simulink model "Diode_Rectifier_Six_Phase_RLload2015"  (R2015b)
settings: Solver=VariableStepAuto  SolverMode=SingleTasking  StartTime=0.0  StopTime=0.04  RelTol=1e-3
undefined symbols (not defined in the file): powergui
libraries: powerlib x24
settings Model: Creator=A.hey  LastModifiedBy=A.hey
settings DataIOCC: LimitDataPoints=off
settings DebuggingCC: AllowSymbolicDim=on  SFUnexpectedBacktrackingDiag=error  SFNoUnconditionalDefaultTransitionDiag=error
settings ModelReferenceCC: PropagateSignalLabelsOutOfModel=on
settings SFSimCC: SimUseLocalCustomCode=on
settings RTWCC: RTWUseLocalCustomCode=on
settings GRTTargetCC: TargetLangStandard=C99 (ISO)
settings ConfigComp: CovMetricSettings=dwe  CovHtmlReporting=off  CovSaveCumulativeToWorkspaceVar=off  CovSaveSingleToWorkspaceVar=off  CovModelRefEnable=Off  CovExternalEMLEnable=on
settings ConfigurationSet: Description=Simscape Multibody

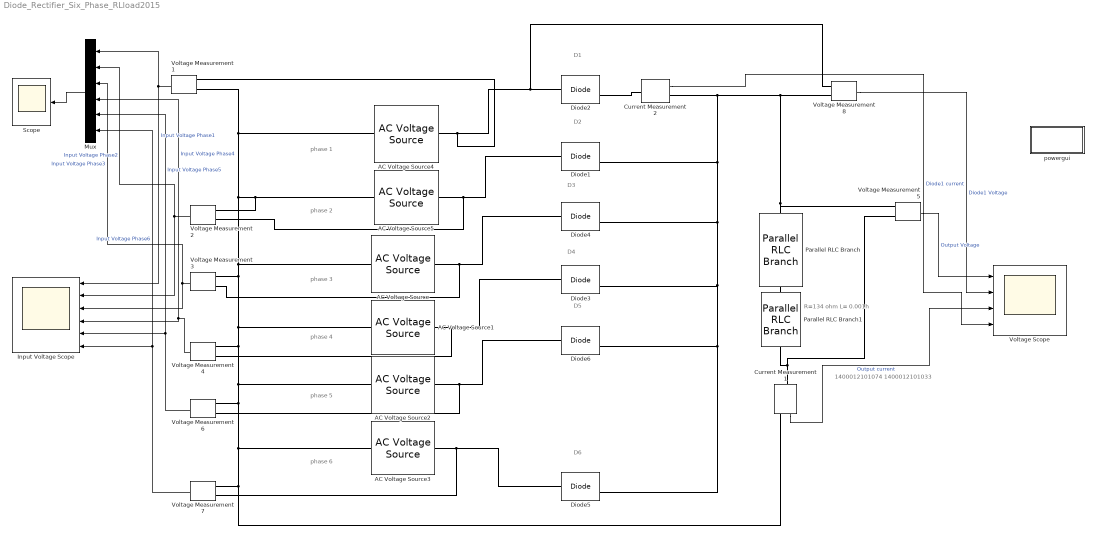
== system Diode_Rectifier_Six_Phase_RLload2015 ==
  note: phase 4
  note: phase 6
  note: phase 1
  note: phase 3
  note: D5
  note: phase 5
  note: D6
  note: D2
  note: phase 2
  note: D1
  note: 1400012101074
      | 1400012101033
  note: D3
  note: D4
  note: R=134 ohm
      | L= 0.001h
  AC Voltage Source : powerlib/Electrical Sources/AC Voltage Source  Amplitude=220  Phase=-180  Frequency=50  SampleTime=0  Measurements=None  BusType=swing  Pref=10e3  Qref=0  Qmin=-inf  Qmax=+inf
  AC Voltage Source1 : powerlib/Electrical Sources/AC Voltage Source  Amplitude=220  Phase=-240  Frequency=50  SampleTime=0  Measurements=None  BusType=swing  Pref=10e3  Qref=0  Qmin=-inf  Qmax=+inf
  AC Voltage Source2 : powerlib/Electrical Sources/AC Voltage Source  Amplitude=220  Phase=-300  Frequency=50  SampleTime=0  Measurements=None  BusType=swing  Pref=10e3  Qref=0  Qmin=-inf  Qmax=+inf
  AC Voltage Source3 : powerlib/Electrical Sources/AC Voltage Source  Amplitude=220  Phase=-360  Frequency=50  SampleTime=0  Measurements=None  BusType=swing  Pref=10e3  Qref=0  Qmin=-inf  Qmax=+inf
  AC Voltage Source4 : powerlib/Electrical Sources/AC Voltage Source  Amplitude=220  Phase=-60  Frequency=50  SampleTime=0  Measurements=None  BusType=swing  Pref=10e3  Qref=0  Qmin=-inf  Qmax=+inf
  AC Voltage Source5 : powerlib/Electrical Sources/AC Voltage Source  Amplitude=220  Phase=-120  Frequency=50  SampleTime=0  Measurements=None  BusType=swing  Pref=10e3  Qref=0  Qmin=-inf  Qmax=+inf
  Current Measurement1 : powerlib/Measurements/Current Measurement  PhasorSimulation=off  OutputType=Complex  PSBequivalent=0
  Current Measurement2 : powerlib/Measurements/Current Measurement  PhasorSimulation=off  OutputType=Complex  PSBequivalent=0
  Diode{1..6} (6 alike) : powerlib/Power Electronics/Diode  Ron=0.001  Lon=0  Vf=0.8  IC=0  UseSnubber=0  Rs=500  Cs=250e-9  Measurements=on
  "Input Voltage Scope " : Scope  NumInputPorts=6
  Mux : Mux  Inputs=6
  Parallel RLC Branch : powerlib/Elements/Parallel RLC Branch  LConnTagsString=a  RConnTagsString=__new0  BranchType=R  Resistance=134  Inductance=1e-3  SetiL0=off  InitialCurrent=0  Capacitance=1e-6  Setx0=off  InitialVoltage=0  Measurements=None
  Parallel RLC Branch1 : powerlib/Elements/Parallel RLC Branch  LConnTagsString=a  RConnTagsString=__new0  BranchType=L  Resistance=134  Inductance=1e-3  SetiL0=off  InitialCurrent=0  Capacitance=1e-6  Setx0=off  InitialVoltage=0  Measurements=None
  Scope : Scope
  Voltage Measurement{1..8} (8 alike) : powerlib/Measurements/Voltage Measurement  PhasorSimulation=off  OutputType=Complex  PSBequivalent=0
  "Voltage Scope " : Scope  NumInputPorts=4
  powergui : Subsystem  Priority=1  AncestorBlock=powerlib/powergui  DialogController=POWERSYS.PowerSysDialog  InitFcn=powergui( 'InitFcn_Callback' , gcb , 0 , [ ] );  mask(PSB option menu block){SimulationMode=Continuous, SampleTime=50e-6, frequency=60, Iterations=50, frequencyindice=50, Pbase=100e6, ErrMax=1e-4, UnitsV=kV, UnitsW=MW, buscounter=0, FunctionMessages=off, echomessages=off, EnableUseOfTLC=off, CurrentSourceSwitches=off, DisableSnubberDevices=off, DisableRonSwitches=off, DisableVfSwitches=off, DisplayEquations=off, SolverType=Tustin/Backward Euler (TBE), Interpol=off, ExternalGateDelay=off, methode=off, Ts=100, x0status=blocks, SPID=on, SwTol=0, HookPort=off, RestoreLinks=warning, ResistiveCurrentMeasurement=off, Frange=[0:2:500], Ylog=off, Xlog=on, ShowGrid=off, save=off, variable=ZData, structure=0, ZoomFFT=off, StartTime=0.0, cycles=1, DisplayStyle=1, fundamental=60, FreqAxis=off, MaxFrequency=1000, frequencyindicesteady=1, RmsSteady=1, display=off}
      mask prompts: SimulationMode "Simulation type:"; SampleTime "Sample time (s):"; frequency "Frequency (Hz):"; Iterations "Max iterations"; frequencyindice "Frequency (Hz)"; Pbase "Base power (VA)"; ErrMax "PQ tolerance (pu)"; UnitsV "Voltage units"; UnitsW "Power units"; buscounter "Load flow bus counter"; FunctionMessages "Disable Specialized Power Systems warnings"; echomessages "Display Specialized Power Systems compilation messages"; EnableUseOfTLC "Use TLC file when in Accelerator Simulation Mode and for code generation"; CurrentSourceSwitches "Disable ideal switching"; DisableSnubberDevices "Disable snubbers in switching devices"; DisableRonSwitches "Disable Ron resistances in switching devices"; DisableVfSwitches "Disable forward voltages in switching devices"; DisplayEquations "Display circuit differential equations"; SolverType "Discrete solver"; Interpol "Interpolate switching events"; ExternalGateDelay "Use time-stamped gate signals"; methode "Store switching topologies"; Ts "Buffer size (MBytes):"; x0status "Start simulation with initial electrical states from:"; SPID "Use ideal switching devices"; SwTol "Switch tolerance"; HookPort "Allow multiple powergui blocks"; RestoreLinks "Restore disabled links of Simscape Power Systems ST blocks:"; ResistiveCurrentMeasurement "Use non ideal current measurement blocks (1e-4Ohm internal resistance)"; Frange "Frequency Range"; Ylog "Log impedance"; Xlog "log Frequency"; ShowGrid "grid"; save "Save Data To Workspace"; variable "Variable Name"; structure "Structure Name (PSBFFTSCOPE)"; ZoomFFT "ZoomFFT (PSBFFTSCOPE)"; StartTime "Start Time (PSBFFTSCOPE)"; cycles "Cycles (PSBFFTSCOPE)"; DisplayStyle "Display style (PSBFFTSCOPE)"; fundamental "Fundamental (PSBFFTSCOPE)"; FreqAxis "Frequency Axis (PSBFFTSCOPE)"; MaxFrequency "Max Frequency (PSBFFTSCOPE)"; frequencyindicesteady "Frequency indice (STEADYSTATE)"; RmsSteady "RMS display (STEADYSTATE)"; display "Display Results"
      mask help: Set simulation type, simulation parameters, and preferences.
      mask init:
      | dispMessage = powergui('MaskInitialization',gcb,SimulationMode,SampleTime);
      settings: PreSaveFcn=powergui( 'PreSaveFcn_Callback' , gcb , [ ] , [ ] );  OpenFcn=sps_rtmsupport('OpenFcn',gcbh)
      mask Help: helpview(psbhelp)
      mask TypeOptions SimulationMode: Continuous | Discrete | Phasor
      mask Callback SimulationMode: powergui('SimulationType',[],[],gcb);
      mask TypeOptions UnitsV: V | kV
      mask TypeOptions UnitsW: W | kW | MW
      mask Callback CurrentSourceSwitches: powergui('SimulationType',[],[],gcb);
      mask TypeOptions SolverType: Tustin/Backward Euler (TBE) | Tustin | Backward Euler
      mask Callback SolverType: powergui('SimulationType',[],[],gcb);
      mask Callback Interpol: powergui('SimulationType',[],[],gcb);
      mask Callback ExternalGateDelay: powergui('SimulationType',[],[],gcb);
      mask Callback methode: powergui('SimulationType',[],[],gcb);
      mask TypeOptions x0status: blocks | steady | zero
      mask TypeOptions RestoreLinks: yes | warning | no
      mask Callback display: sps_rtmsupport('parametereditingmodes',gcbh) % Will be executed last in parameter callbacks to ensure mask enable consistency
      mask DialogControl AutoSolverNote Prompt: To enable the Powergui solver settings, unselect auto (Automatic solver selection) solver in the Simulink solver options.
      mask DialogControl SteadyState Prompt: Steady-State
      mask DialogControl SteadyState Callback: close_system(gcb); power_steadystate(bdroot(gcb),gcb);
      mask DialogControl InitialState Prompt: Initial State
      mask DialogControl InitialState Callback: close_system(gcb); power_initstates(bdroot(gcb),gcb)
      mask DialogControl MachineInitialization Prompt: Machine Initialization
      mask DialogControl MachineInitialization Callback: close_system(gcb); power_loadflow(bdroot(gcb),gcb);
      mask DialogControl ImpedanceMeasurement Prompt: Impedance Measurement
      mask DialogControl ImpedanceMeasurement Callback: close_system(gcb); power_zmeter(bdroot(gcb),gcb);
      mask DialogControl FFTAnalysis Prompt: FFT Analysis
      mask DialogControl FFTAnalysis Callback: close_system(gcb); power_fftscope(bdroot(gcb),gcb);
      mask DialogControl LinearSystemAnalyzer Prompt: Use Linear System Analyzer
      mask DialogControl LinearSystemAnalyzer Callback: close_system(gcb); power_ltiview(bdroot(gcb),gcb);
      mask DialogControl HysteresisDesign Prompt: Hysteresis Design
      mask DialogControl HysteresisDesign Callback: close_system(gcb); power_hysteresis(bdroot(gcb),gcb);
      mask DialogControl RLCLineParameters Prompt: RLC Line Parameters
      mask DialogControl RLCLineParameters Callback: close_system(gcb); power_lineparam(bdroot(gcb),gcb);
      mask DialogControl GenerateReprot Prompt: Generate Report
      mask DialogControl GenerateReprot Callback: close_system(gcb); power_report(bdroot(gcb),gcb);
      mask DialogControl Control14 Prompt: Customize SPS blocks
      mask DialogControl Control14 Callback: close_system(gcb); power_customize;
      mask DialogControl LoadFlow Prompt: Load Flow
      mask DialogControl LoadFlow Callback: close_system(gcb); power_loadflow('-v2',bdroot(gcb));
      mask DialogControl Container14 Prompt: Load flow settings
      mask Display: color('blue'),disp(dispMessage)
  wires:
  Voltage Measurement5/1 -> "Voltage Scope "/1  "Output Voltage"
  Voltage Measurement8/1 -> "Voltage Scope "/2  "Diode1 Voltage"
  Voltage Measurement1/1 -> Mux/1, "Input Voltage Scope "/1  "Input Voltage Phase1"
  Voltage Measurement4/1 -> Mux/4, "Input Voltage Scope "/4  "Input Voltage Phase4"
  Voltage Measurement3/1 -> Mux/3, "Input Voltage Scope "/3  "Input Voltage Phase3"
  Voltage Measurement2/1 -> Mux/2, "Input Voltage Scope "/2  "Input Voltage Phase2"
  Voltage Measurement6/1 -> Mux/5, "Input Voltage Scope "/5  "Input Voltage Phase5"
  Mux/1 -> Scope/1
  Current Measurement2/1 -> "Voltage Scope "/4  "Diode1 current"
  Current Measurement1/1 -> "Voltage Scope "/3  "Output current"
  Voltage Measurement7/1 -> Mux/6, "Input Voltage Scope "/6  "Input Voltage Phase6"
  connections:
  Diode4/RConn1 -- Voltage Measurement8/LConn2 -- Voltage Measurement5/LConn1 -- Parallel RLC Branch/LConn1 -- Current Measurement2/RConn1 -- Diode1/RConn1 -- Diode6/RConn1 -- Diode5/RConn1 -- Diode3/RConn1
  Voltage Measurement7/LConn2 -- Current Measurement1/RConn1 -- AC Voltage Source/LConn1 -- Voltage Measurement1/LConn2 -- AC Voltage Source4/LConn1 -- Voltage Measurement2/LConn2 -- AC Voltage Source5/LConn1 -- Voltage Measurement3/LConn2 -- AC Voltage Source1/LConn1 -- Voltage Measurement4/LConn2 -- AC Voltage Source2/LConn1 -- Voltage Measurement6/LConn2 -- AC Voltage Source3/LConn1
  AC Voltage Source2/RConn1 -- Voltage Measurement6/LConn1 -- Diode6/LConn1
  AC Voltage Source1/RConn1 -- Voltage Measurement4/LConn1 -- Diode3/LConn1
  AC Voltage Source5/RConn1 -- Voltage Measurement2/LConn1 -- Diode1/LConn1
  Voltage Measurement5/LConn2 -- Parallel RLC Branch1/RConn1 -- Current Measurement1/LConn1
  Diode2/LConn1 -- Voltage Measurement8/LConn1 -- Voltage Measurement1/LConn1 -- AC Voltage Source4/RConn1
  AC Voltage Source/RConn1 -- Voltage Measurement3/LConn1 -- Diode4/LConn1
  AC Voltage Source3/RConn1 -- Voltage Measurement7/LConn1 -- Diode5/LConn1
  Current Measurement2/LConn1 -- Diode2/RConn1
  Parallel RLC Branch1/LConn1 -- Parallel RLC Branch/RConn1

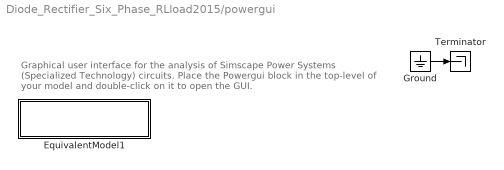
== system Diode_Rectifier_Six_Phase_RLload2015/powergui ==
  note: Graphical user interface for the analysis of
      | Simscape Power Systems (Specialized Technology) circuits.
      | Place the Powergui block in the top-level of your model and double-click
      | on it to open the GUI.
  EquivalentModel1 : Subsystem  mask{SwTol=SwTol}
      mask prompts: SwTol "SwitchTolerance"
      mask init:
      | S  = GetDataForEquivalentModel('SPID',gcbh,SwTol);
      mask Display:
      | color('blue')
      | disp('EQUIVALENT CIRCUIT\nSPID')
  Ground : Ground
  Terminator : Terminator
  wires:
  Ground/1 -> Terminator/1

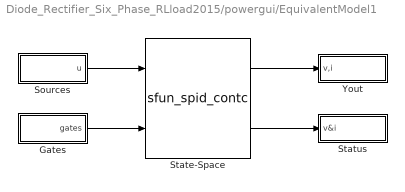
== system Diode_Rectifier_Six_Phase_RLload2015/powergui/EquivalentModel1 ==
  Gates : Subsystem
  Sources : Subsystem
  State-Space : S-Function  FunctionName=sfun_spid_contc  Parameters=S.Mg, [S.nb.x S.nb.u S.nb.y S.nb.s], S.x0, S.MgColNames, S.SwitchVf, S.SwitchType, S.SwitchGateInitialValue, S.SwitchTolerance,S.SaveMatrices,S.BufferSize  SFunctionDeploymentMode=off  EnableBusSupport=off
  Status : Subsystem
  Yout : Subsystem
  wires:
  State-Space/1 -> Yout/1(v,i)
  State-Space/2 -> Status/1(v&i)
  Gates/1(gates) -> State-Space/2
  Sources/1(u) -> State-Space/1

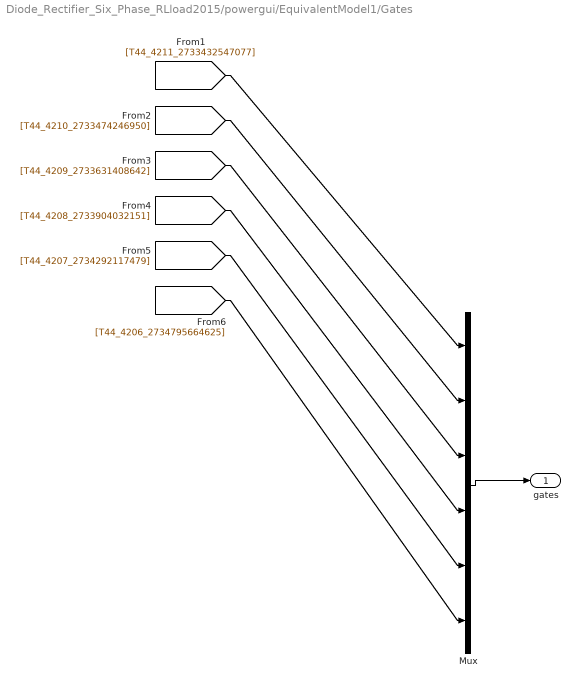
== system Diode_Rectifier_Six_Phase_RLload2015/powergui/EquivalentModel1/Gates ==
  Mux : Mux  Inputs=[1 1 1 1 1 1]
  gates : Outport
  wires:
  Mux/1 -> gates/1
  [T44_4211_2733432547077] -> Mux/1
  [T44_4210_2733474246950] -> Mux/2
  [T44_4209_2733631408642] -> Mux/3
  [T44_4208_2733904032151] -> Mux/4
  [T44_4207_2734292117479] -> Mux/5
  [T44_4206_2734795664625] -> Mux/6

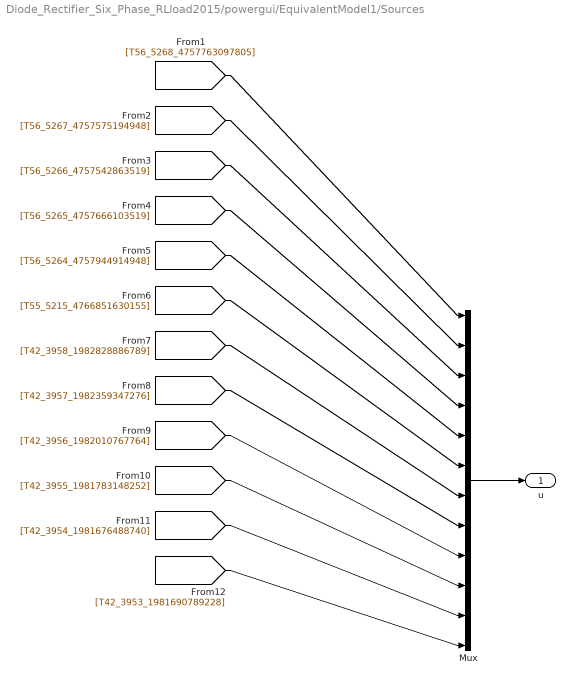
== system Diode_Rectifier_Six_Phase_RLload2015/powergui/EquivalentModel1/Sources ==
  Mux : Mux  Inputs=[1 1 1 1 1 1 1 1 1 1 1 1]
  u : Outport
  wires:
  Mux/1 -> u/1
  [T56_5268_4757763097805] -> Mux/1
  [T56_5267_4757575194948] -> Mux/2
  [T56_5266_4757542863519] -> Mux/3
  [T56_5265_4757666103519] -> Mux/4
  [T56_5264_4757944914948] -> Mux/5
  [T55_5215_4766851630155] -> Mux/6
  [T42_3958_1982828886789] -> Mux/7
  [T42_3957_1982359347276] -> Mux/8
  [T42_3956_1982010767764] -> Mux/9
  [T42_3955_1981783148252] -> Mux/10
  [T42_3954_1981676488740] -> Mux/11
  [T42_3953_1981690789228] -> Mux/12

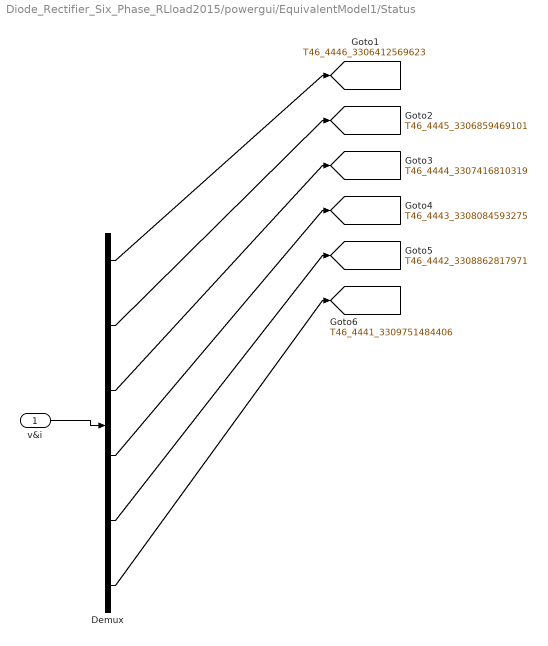
== system Diode_Rectifier_Six_Phase_RLload2015/powergui/EquivalentModel1/Status ==
  v&i : Inport
  Demux : Demux  Outputs=[2 2 2 2 2 2]
  tag scope: T46_4441_3309751484406=global, T46_4442_3308862817971=global, T46_4443_3308084593275=global, T46_4444_3307416810319=global, T46_4445_3306859469101=global, T46_4446_3306412569623=global
  wires:
  v&i/1 -> Demux/1
  Demux/1 -> [T46_4446_3306412569623]
  Demux/2 -> [T46_4445_3306859469101]
  Demux/3 -> [T46_4444_3307416810319]
  Demux/4 -> [T46_4443_3308084593275]
  Demux/5 -> [T46_4442_3308862817971]
  Demux/6 -> [T46_4441_3309751484406]

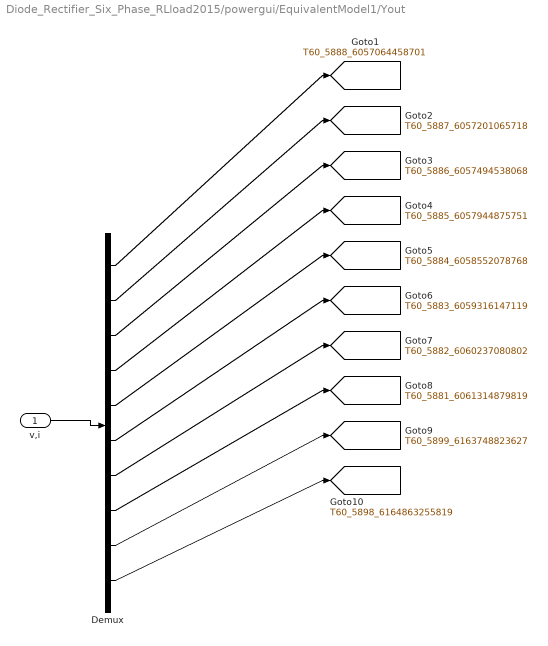
== system Diode_Rectifier_Six_Phase_RLload2015/powergui/EquivalentModel1/Yout ==
  v,i : Inport
  Demux : Demux  Outputs=[1 1 1 1 1 1 1 1 1 1]
  tag scope: T60_5881_6061314879819=global, T60_5882_6060237080802=global, T60_5883_6059316147119=global, T60_5884_6058552078768=global, T60_5885_6057944875751=global, T60_5886_6057494538068=global, T60_5887_6057201065718=global, T60_5888_6057064458701=global, T60_5898_6164863255819=global, T60_5899_6163748823627=global
  wires:
  v,i/1 -> Demux/1
  Demux/1 -> [T60_5888_6057064458701]
  Demux/2 -> [T60_5887_6057201065718]
  Demux/3 -> [T60_5886_6057494538068]
  Demux/4 -> [T60_5885_6057944875751]
  Demux/5 -> [T60_5884_6058552078768]
  Demux/6 -> [T60_5883_6059316147119]
  Demux/7 -> [T60_5882_6060237080802]
  Demux/8 -> [T60_5881_6061314879819]
  Demux/9 -> [T60_5899_6163748823627]
  Demux/10 -> [T60_5898_6164863255819]
